simulink model "NonLinearVehicleiLQR"  (R2021a)
settings: Solver=FixedStepDiscrete  StartTime=0.0  StopTime=100  FixedStep=0.001  MaxStep=0.01  RelTol=1e-3
values from neighbouring files (symbols this model uses):
  L = 0.189    [NonlinearVehicleLQR.m]    (also in NonlinearVehicleiLQR.m; linearVehicleiLQR.m)
  Q = [1 0 0; 0 1 0; 0 0 10]    [LQR.m]    (also in NonlinearVehicleLQR.m = eye(3)*10; NonlinearVehicleiLQR.m = eye(3)*10; SringiLQR.m = [1 0; 0 1]*1; SringiLQR2.m = [1 0; 0 1]*1)
  Qf = eye(3)    [LQR.m]    (also in NonlinearVehicleLQR.m; NonlinearVehicleiLQR.m; SringiLQR.m = [1 0; 0 1]; SringiLQR2.m = [1 0; 0 1])
  R = eye(2)*10^-4    [LQR.m]    (also in NonlinearVehicleLQR.m = eye(2)*10^-2; NonlinearVehicleiLQR.m = eye(2)*10^-2; SringiLQR.m = eye(1)*1e-2; SringiLQR2.m = eye(1)*1e-2)
  Radius = 0.02    [NonlinearVehicleLQR.m]    (also in NonlinearVehicleiLQR.m; linearVehicleiLQR.m)
undefined symbols (not defined in the file or in its folder): DiscIntNeverNeededParam
settings Model: Creator=iris  LastModifiedBy=iris
settings SolverCC: AlgebraicLoopSolver=TrustRegion
settings DebuggingCC: SFMachineParentedDataDiag=warning

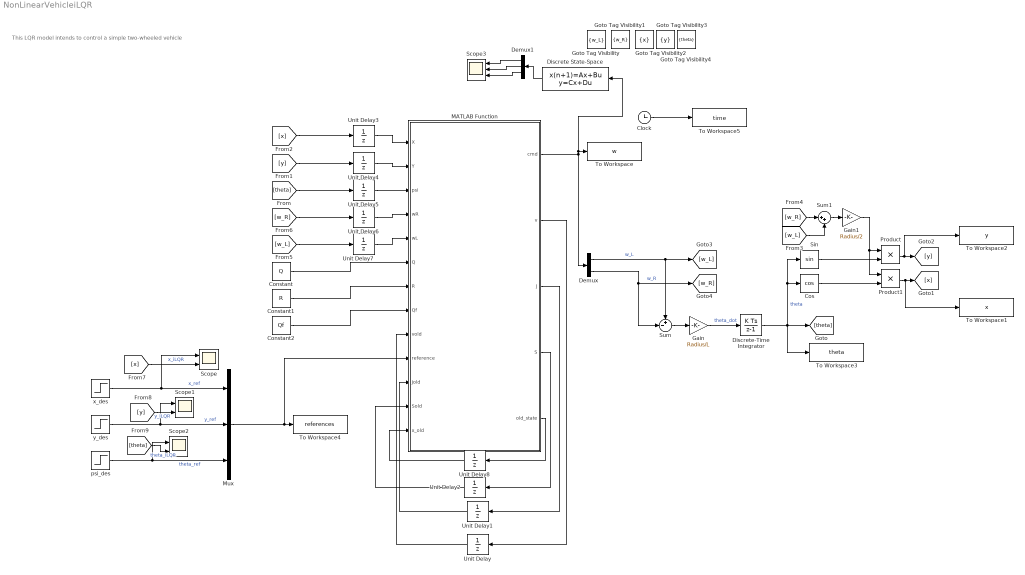
== system NonLinearVehicleiLQR ==
  note: This LQR model intends to control a simple two-wheeled vehicle
  Clock : Clock
  Constant : Constant  Value=Q
  Constant1 : Constant  Value=R
  Constant2 : Constant  Value=Qf
  Cos : Trigonometry  Operator=cos
  Demux : Demux  Outputs=2
  Demux1 : Demux  Outputs=3
  Discrete State-Space : DiscreteStateSpace  A=eye(3)  B=[0.001 0;0 0; 0 0.001]  C=eye(3)  D=zeros(3,2)  SampleTime=-1
  Discrete-Time Integrator : DiscreteIntegrator  SampleTime=-1  ICPrevOutput=DiscIntNeverNeededParam  ICPrevScaledInput=DiscIntNeverNeededParam
  Gain : Gain  Gain=Radius/L
  Gain1 : Gain  Gain=Radius/2
  Goto Tag Visibility : GotoTagVisibility  GotoTag=w_L
  Goto Tag Visibility1 : GotoTagVisibility  GotoTag=w_R
  Goto Tag Visibility2 : GotoTagVisibility  GotoTag=x
  Goto Tag Visibility3 : GotoTagVisibility  GotoTag=y
  Goto Tag Visibility4 : GotoTagVisibility  GotoTag=theta
  MATLAB Function : MATLAB Function  TreatAsAtomicUnit=on
  Mux : Mux  Inputs=3
  Product : Product
  Product1 : Product
  Scope : Scope  NumInputPorts=2
  Scope1 : Scope  NumInputPorts=2
  Scope2 : Scope  NumInputPorts=2
  Scope3 : Scope  NumInputPorts=3
  Sin : Trigonometry
  Sum : Sum  Inputs=+-|
  Sum1 : Sum  Inputs=|++
  To Workspace : ToWorkspace  VariableName=w  SampleTime=-1
  To Workspace1 : ToWorkspace  VariableName=x  SampleTime=-1
  To Workspace2 : ToWorkspace  VariableName=y  SampleTime=-1
  To Workspace3 : ToWorkspace  VariableName=theta  SampleTime=-1
  To Workspace4 : ToWorkspace  VariableName=references  SampleTime=-1
  To Workspace5 : ToWorkspace  VariableName=time  SampleTime=-1
  Unit Delay : UnitDelay  InitialCondition=zeros(3,1)  SampleTime=-1  HasFrameUpgradeWarning=on
  Unit Delay1 : UnitDelay  InitialCondition=10000  SampleTime=-1  HasFrameUpgradeWarning=on
  Unit Delay2 : UnitDelay  InitialCondition=Qf  SampleTime=-1  HasFrameUpgradeWarning=on
  Unit Delay{3..7} (5 alike) : UnitDelay  SampleTime=-1  HasFrameUpgradeWarning=on
  Unit Delay8 : UnitDelay  InitialCondition=[0,0,0]  SampleTime=-1  HasFrameUpgradeWarning=on
  psi_des : Step  Time=0  After=0  SampleTime=0
  x_des : Step  Time=0  SampleTime=0
  y_des : Step  Time=0  After=0  SampleTime=0
  wires:
  MATLAB Function/3(J) -> Unit Delay1/1
  Unit Delay1/1 -> MATLAB Function/11(Jold)
  MATLAB Function/4(S) -> Unit Delay2/1
  Unit Delay2/1 -> MATLAB Function/12(Sold)
  MATLAB Function/2(v) -> Unit Delay/1
  Unit Delay/1 -> MATLAB Function/9(vold)
  MATLAB Function/1(cmd) -> Demux/1, Discrete State-Space/1, To Workspace/1
  Demux/1 -> [w_L], Sum/1  "w_L"
  Demux/2 -> Sum/2, [w_R]  "w_R"
  Sum/1 -> Gain/1
  Gain/1 -> Discrete-Time Integrator/1  "theta_dot"
  Discrete-Time Integrator/1 -> [theta], To Workspace3/1, Sin/1, Cos/1  "theta"
  [theta] -> Unit Delay5/1
  [x] -> Unit Delay3/1
  [y] -> Unit Delay4/1
  [w_R] -> Sum1/1
  [w_L] -> Sum1/2
  Cos/1 -> Product1/2
  Sin/1 -> Product/2
  Sum1/1 -> Gain1/1
  Gain1/1 -> Product1/1, Product/1
  Product1/1 -> To Workspace1/1, [x]
  Product/1 -> To Workspace2/1, [y]
  [w_L] -> Unit Delay7/1
  [w_R] -> Unit Delay6/1
  Constant/1 -> MATLAB Function/6(Q)
  Constant1/1 -> MATLAB Function/7(R)
  Constant2/1 -> MATLAB Function/8(Qf)
  Mux/1 -> MATLAB Function/10(reference), To Workspace4/1
  y_des/1 -> Scope1/1, Mux/2  "y_ref"
  x_des/1 -> Mux/1, Scope/1  "x_ref"
  psi_des/1 -> Scope2/1, Mux/3  "theta_ref"
  Unit Delay3/1 -> MATLAB Function/1(X)
  Unit Delay4/1 -> MATLAB Function/2(Y)
  Unit Delay5/1 -> MATLAB Function/3(psi)
  Unit Delay6/1 -> MATLAB Function/4(wR)
  Unit Delay7/1 -> MATLAB Function/5(wL)
  Clock/1 -> To Workspace5/1
  [x] -> Scope/2  "x_iLQR"
  [y] -> Scope1/2  "y_iLQR"
  [theta] -> Scope2/2  "theta_iLQR"
  Discrete State-Space/1 -> Demux1/1
  Demux1/1 -> Scope3/1
  Demux1/3 -> Scope3/3
  Demux1/2 -> Scope3/2
  MATLAB Function/5(old_state) -> Unit Delay8/1
  Unit Delay8/1 -> MATLAB Function/13(x_old)

== matlab function NonLinearVehicleiLQR/MATLAB Function ==
  data: X input; cmd output; Y input; psi input; wR input; wL input; Q input; R input; Qf input; vold input; reference input; Jold input; Sold input; v output; J output; S output; old_state output; x_old input
function [cmd, v, J, S, old_state]= fcn(X, Y, psi, wR, wL, Q, R, Qf, vold, reference, Jold, Sold, x_old)

r = 0.02;
B = 0.185;
dt = 0.001;

% toll = 3*10^-5;

% A = [1 0 dt*-sin(psi)*r/2*(wR+wL);...
%      0 1 dt*cos(psi)*r/2*(wR+wL);...
%      0 0 1];
% B = dt*[cos(psi)*r/2 cos(psi)*r/2;...
%      sin(psi)*r/2 sin(psi)*r/2;...
%      -r/B r/B];
% A = eye(3);
% B = dt*[1 0;...
%      0 0;...
%      0 1];
A = [1 0 dt*-sin(psi)*r/2*(wR+wL);...
     0 1 dt*cos(psi)*r/2*(wR+wL);...
     0 0 1];
B = dt*[cos(psi)*r/2 cos(psi)*r/2;...
     sin(psi)*r/2 sin(psi)*r/2;...
     -r/B r/B];
state = [X Y psi];
cmd_old = [wL wR];
J = state*Qf*state'+state*Q*state'+cmd_old*R*cmd_old';


% if abs(Jold-J)/Jold > toll
K  = (B'*Sold*B+R)\B'*Sold*A;
Kv = (B'*Sold*B+R)\B';
Ku = (B'*Sold*B+R)\R;
S  = A'*Sold*(A-B*K)+Q;
deltax = -reference;
v  = (A-B*K)'*vold-K'*R*cmd_old'+Q*deltax;

deltau = -K*(x_old'-state)'-Kv*v-Ku*cmd_old';
old_state = state';
cmd  = cmd_old' + deltau;
% else
%     S  = Sold;
%     v  = vold;
%     cmd  = [wL wR]';
end
